simulink model "TimeResponseExperiment"  (R2023a)
settings: Solver=FixedStepDiscrete  StartTime=0.0  StopTime=5  FixedStep=0.01  RelTol=1e-3  EnableMultiTasking=on
libraries: M5Core_Library x2, eeGeneralControl x1
settings Model: ExtModeTrigDuration=2  Creator=auw_a  LastModifiedBy=auw_a
settings OptimizationCC: EnhancedBackFolding=on  PassReuseOutputArgsAs=Individual arguments  ZeroExternalMemoryAtStartup=off  ZeroInternalMemoryAtStartup=off  MaxStackSize=64  OptimizeBlockOrder=speed  DifferentSizesBufferReuse=on  OptimizationCustomize=off  EfficientTunableParamExpr=on
settings DebuggingCC: ParameterOverflowMsg=none  ParameterTunabilityLossMsg=error
settings HardwareCC: ProdBitPerPointer=32  ProdBitPerSizeT=32  ProdBitPerPtrDiffT=32  ProdLargestAtomicInteger=Long  ProdLargestAtomicFloat=Double  ProdWordSize=32  ProdHWDeviceType=ARM Compatible->ARM Cortex
settings SFSimCC: MATLABDynamicMemAlloc=off
settings RTWCC: Description=Embedded Coder  SystemTargetFile=ert.tlc  HardwareBoard=ESP32-WROOM(Arduino Compatible)  TLCOptions="-aInlineSetEventsForThisBaseRateFcn=TLC_FALSE -aSuppressMultiTaskScheduler=TLC_FALSE  -aRateBasedStepFcn=0"  TemplateMakefile=ert_default_tmf  Toolchain=ESP32  BuildConfiguration=Faster Runs
settings CodeAppCC: ForceParamTrailComments=on  IgnoreCustomStorageClasses=off  OperatorAnnotations=on  SimulinkDataObjDesc=on  SFDataObjDesc=on  InsertBlockDesc=on
settings ERTTargetCC: SupportContinuousTime=on  SupportVariableSizeSignals=on  ExtModeTransport=3  ExtModeStaticAlloc=on  ExtModeAutomaticAllocSize=off  ExtModeStaticAllocSize=65536  ExtModeMexFile=ext_xcp  ExtModeIntrfLevel=Level2 - Open

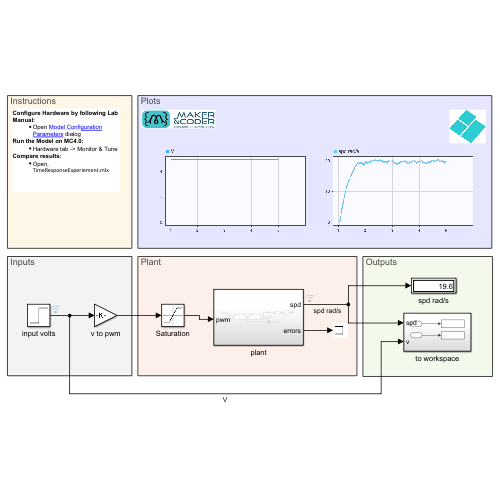
[thumbnail: Simulink's stored preview of the top-level diagram]
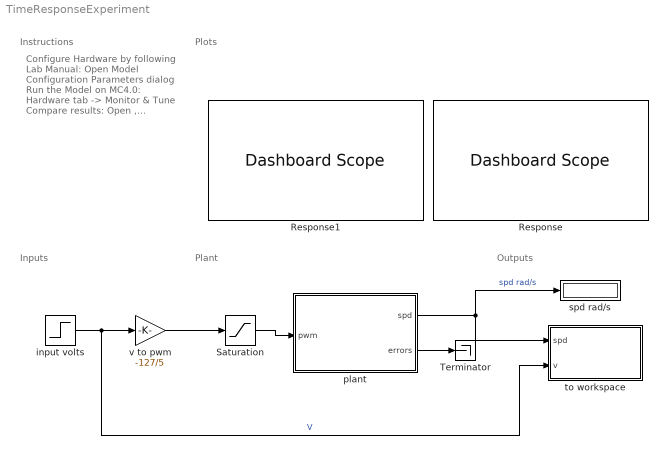
== system TimeResponseExperiment ==
  note: Configure Hardware by following Lab Manual:
      | Open Model Configuration Parameters dialog
      | Run the Model on MC4.0:
      | Hardware tab -> Monitor & Tune
      | Compare results:
      | Open , TimeResponseExperiement.mlx
  note: Instructions
  note: Outputs
  note: Plots
  note: Inputs
  note: Plant
  Response : DashboardScope  Ymin=0  Ymax=5  UpdateMode=Scroll
  Response1 : DashboardScope  Ymin=0  Ymax=6  UpdateMode=Scroll
  Saturation : Saturate  UpperLimit=127  LowerLimit=-127  OutDataTypeStr=int8
  Terminator : Terminator
  input volts : Step  After=5  SampleTime=0.01
  plant : Subsystem
  spd rad/s : Display
  to workspace : Subsystem
  v to pwm : Gain  Gain=-127/5
  wires:
  Saturation/1 -> plant/1(pwm)
  v to pwm/1 -> Saturation/1
  input volts/1 -> to workspace/2(v), v to pwm/1  "V"
  plant/2(errors) -> Terminator/1
  plant/1(spd) -> to workspace/1(spd), spd rad/s/1  "spd rad/s"

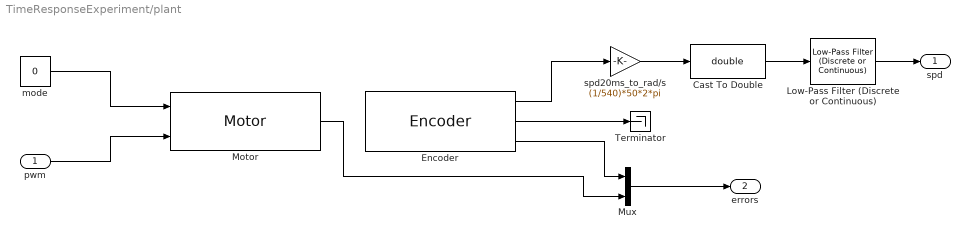
== system TimeResponseExperiment/plant ==
  pwm : Inport
  Cast To Double : DataTypeConversion  OutDataTypeStr=double  SaturateOnIntegerOverflow=off  RndMeth=Floor
  Encoder : M5Core_Library/Encoder  M5_motor=2  s=0.01
  Low-Pass Filter (Discrete or Continuous) : eeGeneralControl/Low-Pass Filter (Discrete or Continuous)  K=1  T=0.25  B=inf  A=-inf  init_option=Inherited from block input  x0=0  Ts=-1
  Motor : M5Core_Library/Motor  M5_motor=M2
  Mux : Mux  Inputs=2
  Terminator : Terminator
  mode : Constant  Value=0
  spd20ms_to_rad/s : Gain  Gain=(1/540)*50*2*pi
  spd : Outport
  errors : Outport  Port=2
  wires:
  Mux/1 -> errors/1
  mode/1 -> Motor/1
  pwm/1 -> Motor/2
  Motor/1 -> Mux/2
  Encoder/3 -> Mux/1
  Encoder/2 -> Terminator/1
  Cast To Double/1 -> Low-Pass Filter (Discrete or Continuous)/1
  spd20ms_to_rad/s/1 -> Cast To Double/1
  Encoder/1 -> spd20ms_to_rad/s/1
  Low-Pass Filter (Discrete or Continuous)/1 -> spd/1

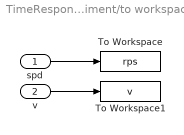
== system TimeResponseExperiment/to workspace ==
  spd : Inport
  v : Inport  Port=2
  To Workspace : ToWorkspace  VariableName=rps  SampleTime=-1
      settings: Save2DSignal=2-D array (concatenate along first dimension)
  To Workspace1 : ToWorkspace  VariableName=v  SampleTime=-1
      settings: Save2DSignal=2-D array (concatenate along first dimension)
  wires:
  spd/1 -> To Workspace/1
  v/1 -> To Workspace1/1
